simulink model "SimpleVAV"  (R2020a)
settings: Solver=FixedStepAuto  StartTime=0.0  StopTime=7200  RelTol=1e-3
settings Model: Creator=yangyang.fu  LastModifiedBy=yangyang.fu

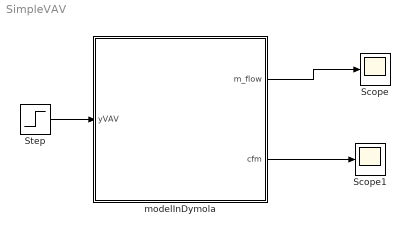
== system SimpleVAV ==
  Scope : Scope
  Scope1 : Scope
  Step : Step  Time=3600  Before=0.5  SampleTime=0.1
  modelInDymola : Subsystem  Tag=07-Sep-2021 15:10:03#975
      mask help:
      | Dymola block.
      | A dymola block allows acausal physical modeling.
      | See Dymola manual for usage.
      settings: CopyFcn=newDymolaGui('07-Sep-2021 15:10:03#975','Copy');  DeleteFcn=if exist('newDymolaGui') newDymolaGui('SimpleVAV/modelInDymola','Delete'); end;  NameChangeFcn=newDymolaGui('07-Sep-2021 15:10:03#975','Copy');  OpenFcn=newDymolaGui('SimpleVAV/modelInDymola','Init');
      mask Display: image(reshape([1;1;1;1;1;1;1;1;1;1;1;1;1;1;1;1;1;1;1;1;1;1;0;0;0;0;0;0;0;0;0;0;1;1;1;1;1;1;1;1;0;1;1;1;1;1;1;1;1;0;1;1;1;1;1;0;0;0;0;0;0;0;1;1;0;0;0;0;0;0;0;1;1;0;0;0;0;0;0;0;1;1;0;0;0;0;0;0;0;1;1;0;0;0;0;0;0;0;1;1;0;0;0;0;0;0;0;1;1;0;0;0;0;0;0;0;1;1;0;0;0;0;0;0;0;1;1;0;0;0;0;0;0;0;1;1;0;0;0;0;0;0;0;1;1;0;0;0;0;0;0;0;1;1;0;0;0;0;0;0;0;1;1;0;0;0;0;0;0;0;1;1;0;0;0;0;0;0;0;1;1;0;0;0;0;0;0;0;1;1;0;0;0;0;0;0;0;1;1;0;0;0;0;0;0;0;1;1;0;0;0;0;0;0;0;1;1;0;0;0;0;0;0;0;1;1;0;0;0;0;0;0;0;1;1;0;0;0;0;0;0;0;1;1;0;0;0;0;0;0;0;1;1;0;0;0;0;0;0;0;1;1;0;0;0;0;0;0;0;1;1;1;1;1;0;1;1;1;1;1;1;1;1;0;1;1;1;1;1;1;1;1;0;0;0;0;0;0;0;0;0;0;1;1;1;1;1;1;1;1;1;1;1;1;1;1;1;1;1;1;1;1;1;1;1;1;1;1;1;1;1;1;1;1;1;1;1;1;1;1;1;1;1;1;1;1;0;0;0;0;0;0;0;0;0;0;1;1;1;1;1;1;1;1;0;1;1;1;1;1;1;1;1;0;1;1;1;1;1;0;0;0;0;0;0;0;1;1;0;0;0;0;0;0;0;1;1;0;0;0;0;0;0;0;1;1;0;0;0;0;0;0;0;1;1;0;0;0;0;0;0;0;1;1;0;0;0;0;0;0;0;1;1;0;0;0;0;0;0;0;1;1;0;0;0;0;0;0;0;1;1;0;0;0;0;0;0;0;1;1;0;0;0;0;0;0;0;1;1;0;0;0;0;0;0;0;1;1;0;0;0;0;0;0;0;1;1;0;0;0;0;0;0;0;1;1;0;0;0;0;0;0;0;1;1;0;0;0;0;0;0;0;1;1;0;0;0;0;0;0;0;1;1;0;0;0;0;0;0;0;1;1;0;0;0;0;0;0;0;1;1;0;0;0;0;0;0;0;1;1;0;0;0;0;0;0;0;1;1;0;0;0;0;0;0;0;1;1;0;0;0;0;0;0;0;1;1;0;0;0;0;0;0;0;1;1;0;0;0;0;0;0;0;1;1;1;1;1;0;1;1;1;1;1;1;1;1;0;1;1;1;1;1;1;1;1;0;0;0;0;0;0;0;0;0;0;1;1;1;1;1;1;1;1;1;1;1;1;1;1;1;1;1;1;1;1;1;1;1;1;1;1;1;1;1;1;1;1;1;1;1;1;1;1;1;1;1;1;1;1;0;0;0;0;0;0;0;0;0;0;1;1;1;1;1;1;1;1;0;1;1;1;1;1;1;1;1;0;1;1;1;1;1;0;0;0;0;0;0;0;1;1;0;0;0;0;0;0;0;1;1;0;1;1;1;1;1;0;1;1;0;1;1;1;1;1;0;1;1;0;1;1;1;1;1;0;1;1;0;1;1;1;1;1;0;1;1;0;1;1;1;1;1;0;1;1;0;1;1;1;1;1;0;1;1;0;1;1;1;1;1;0;1;1;0;1;1;1;1;1;0;1;1;0;1;1;1;1;1;0;1;1;0;1;1;1;1;1;0;1;1;0;1;1;1;1;1;0;1;1;0;1;1;1;1;1;0;1;1;0;1;1;1;1;1;0;1;1;0;1;1;1;1;1;0;1;1;0;1;1;1;1;1;0;1;1;0;1;1;1;1;1;0;1;1;0;1;1;1;1;1;0;1;1;0;1;1;1;1;1;0;1;1;0;1;1;1;1;1;0;1;1;0;1;1;1;1;1;0;1;1;0;0;0;0;0;0;0;1;1;0;0;0;0;0;0;0;1;1;1;1;1;0;1;1;1;1;1;1;1;1;0;1;1;1;1;1;1;1;1;0;0;0;0;0;0;0;0;0;0;1;1;1;1;1;1;1;1;1;1;1;1;1;1;1;1;1;1;1;1;1;1],18,18,3),[.2,.2,.6,.6])
  wires:
  Step/1 -> modelInDymola/1(yVAV)
  modelInDymola/1(m_flow) -> Scope/1
  modelInDymola/2(cfm) -> Scope1/1

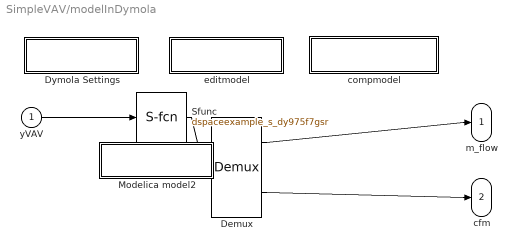
== system SimpleVAV/modelInDymola ==
  yVAV : Inport
  Demux : Demux  Outputs=[1;1]
  Dymola Settings : Subsystem  mask{ModelName=dSpaceExample.SimpleVAV, MoFileName=D:/github/dspace-modelica-example/dSpaceExample/SimpleVAV.mo, dSpace=, BusConnector=[], ResultFile=[], ResultFileOnline=[], ResultDt=[], Libs=:, bigobj=[], ImportFolder=[], guimode=[], ModelName2=[], forRuntime=[], MEXLoad=[], omitDescription=[], ResultName=dspaceexample_s_dy975f7gsr}
      mask prompts: ModelName "Name of Dymola model"; MoFileName "File Name (including .mo)"; ResultFile "Create Result"; ResultFileOnline "Load result"; ResultDt "Result min dt"; Libs "Used Libraries"; bigobj "Compiler flag /bigobj"; ImportFolder "Import folder"; guimode "GUI mode flag"; ModelName2 "Model name for import mode"; forRuntime "Runtime export"; MEXLoad "Compiled S-function"; omitDescription "Omit description strings"; ResultName "Name of result file"
      mask Display: disp('Dymola Settings');
  Modelica model2 : Subsystem
      mask Display: disp('Change parameters');
  Sfunc : S-Function  Tag=975f7gsr  FunctionName=dspaceexample_s_dy975f7gsr  Parameters=[vav_vav_sta_default_p;vav_vav_sta_default_T;vav_vav_sta_default_X;vav_vav_riseTime;vav_vav_y_start;vav_vav_filter_gain;vav_vav_filter_A_ripple;vav_vav_filter_f_min;vav_vav_filter_normalized;vav_vav_filter_x_start;vav_vav_filter_u_nominal;vav_vav_use_deltaM;vav_vav_deltaM;vav_vav_roundDuct;vav_vav_ReC;vav_vav_a;vav_vav_b;vav_vav_yL;vav_vav_yU;vav_vav_k1;vav_vav_l;vav_vav_l2;vav_vav_deltax;vav_vav_y_min;vav_terHea_bal1_preDro_st25;vav_terHea_bal1_preDro_st26;vav_terHea_bal1_preDro_st27;vav_terHea_bal2_preDro_st28;vav_terHea_bal2_preDro_st29;vav_terHea_delta;vav_terHea_T_a1_nominal;vav_terHea_T_a2_nominal;vav_terHea_r_nominal;vav_terHea_hA_n_w;vav_terHea_hA_n_a;vav_terHea_hA_T0_w;vav_terHea_hA_T0_a;vav_sinTer_X;vav_sinTer_p;vav_sinTer_T;vav_souTer_X;vav_souTer_m_flow;vav_souTer_T;zer_k;sou_X;sou_p;sou_T;sin_X;sin_p;sin_T;VRoo;toVol_k],[vav_vav_filter_x]  PortCounts=[1;1]  SFunctionDeploymentMode=off  EnableBusSupport=off  mask{vav_vav_sta_default_p=101325, vav_vav_sta_default_T=293.15, vav_vav_sta_default_X=[0.01; 0.99], vav_vav_riseTime=120, vav_vav_y_start=1, vav_vav_filter_gain=1, vav_vav_filter_A_ripple=0.5, vav_vav_filter_f_min=0, vav_vav_filter_normalized=1, vav_vav_filter_x_start=[0; 0], vav_vav_filter_u_nominal=1, vav_vav_use_deltaM=1, vav_vav_deltaM=0.3, vav_vav_roundDuct=0, vav_vav_ReC=4000, vav_vav_a=-1.51, vav_vav_b=9.45, vav_vav_yL=0.166666666666667, vav_vav_yU=0.611111111111111, vav_vav_k1=0.45, vav_vav_l=0.0001, vav_vav_l2=0.01, vav_vav_deltax=0.02, vav_vav_y_min=0.02, vav_terHea_bal1_preDro_st25=101325, vav_terHea_bal1_preDro_st26=293.15, vav_terHea_bal1_preDro_st27=[0.01; 0.99], vav_terHea_bal2_preDro_st28=300000, vav_terHea_bal2_preDro_st29=293.15, vav_terHea_delta=0.001, vav_terHea_T_a1_nominal=289.85, vav_terHea_T_a2_nominal=355.35, vav_terHea_r_nominal=0.666666666666667, vav_terHea_hA_n_w=0.85, vav_terHea_hA_n_a=0.8, vav_terHea_hA_T0_w=293.15, vav_terHea_hA_T0_a=293.15, vav_sinTer_X=1, vav_sinTer_p=300000, vav_sinTer_T=293.15, vav_souTer_X=1, vav_souTer_m_flow=0, vav_souTer_T=323.15, zer_k=0, sou_X=[0.01; 0.99], sou_p=101565, sou_T=286.15, sin_X=[0.01; 0.99], sin_p=101325, sin_T=293.15, VRoo=2698, toVol_k=1642.54263565891, vav_vav_filter_x=[0; 0]}
      mask prompts: vav_vav_sta_default_p "vav.vav.sta_default.p"; vav_vav_sta_default_T "vav.vav.sta_default.T"; vav_vav_sta_default_X "vav.vav.sta_default.X"; vav_vav_riseTime "vav.vav.riseTime"; vav_vav_y_start "vav.vav.y_start"; vav_vav_filter_gain "vav.vav.filter.gain"; vav_vav_filter_A_ripple "vav.vav.filter.A_ripple"; vav_vav_filter_f_min "vav.vav.filter.f_min"; vav_vav_filter_normalized "vav.vav.filter.normalized"; vav_vav_filter_x_start "vav.vav.filter.x_start"; vav_vav_filter_u_nominal "vav.vav.filter.u_nominal"; vav_vav_use_deltaM "vav.vav.use_deltaM"; vav_vav_deltaM "vav.vav.deltaM"; vav_vav_roundDuct "vav.vav.roundDuct"; vav_vav_ReC "vav.vav.ReC"; vav_vav_a "vav.vav.a"; vav_vav_b "vav.vav.b"; vav_vav_yL "vav.vav.yL"; vav_vav_yU "vav.vav.yU"; vav_vav_k1 "vav.vav.k1"; vav_vav_l "vav.vav.l"; vav_vav_l2 "vav.vav.l2"; vav_vav_deltax "vav.vav.deltax"; vav_vav_y_min "vav.vav.y_min"; vav_terHea_bal1_preDro_st25 "vav.terHea.bal1.preDro.sta_default.p"; vav_terHea_bal1_preDro_st26 "vav.terHea.bal1.preDro.sta_default.T"; vav_terHea_bal1_preDro_st27 "vav.terHea.bal1.preDro.sta_default.X"; vav_terHea_bal2_preDro_st28 "vav.terHea.bal2.preDro.sta_default.p"; vav_terHea_bal2_preDro_st29 "vav.terHea.bal2.preDro.sta_default.T"; vav_terHea_delta "vav.terHea.delta"; vav_terHea_T_a1_nominal "vav.terHea.T_a1_nominal"; vav_terHea_T_a2_nominal "vav.terHea.T_a2_nominal"; vav_terHea_r_nominal "vav.terHea.r_nominal"; vav_terHea_hA_n_w "vav.terHea.hA.n_w"; vav_terHea_hA_n_a "vav.terHea.hA.n_a"; vav_terHea_hA_T0_w "vav.terHea.hA.T0_w"; vav_terHea_hA_T0_a "vav.terHea.hA.T0_a"; vav_sinTer_X "vav.sinTer.X"; vav_sinTer_p "vav.sinTer.p"; vav_sinTer_T "vav.sinTer.T"; vav_souTer_X "vav.souTer.X"; vav_souTer_m_flow "vav.souTer.m_flow"; vav_souTer_T "vav.souTer.T"; zer_k "zer.k"; sou_X "sou.X"; sou_p "sou.p"; sou_T "sou.T"; sin_X "sin.X"; sin_p "sin.p"; sin_T "sin.T"; toVol_k "toVol.k"; vav_vav_filter_x "vav.vav.filter.x"
      mask Display: image(imread('Dymola.bmp'))
  compmodel : Subsystem
      settings: OpenFcn=compileModelica('SimpleVAV/modelInDymola');
      mask Display: disp('Compile Modelica model');
  editmodel : Subsystem
      settings: OpenFcn=editModelica('SimpleVAV/modelInDymola');
      mask Display: disp('Edit Modelica model');
  m_flow : Outport
  cfm : Outport  Port=2
  wires:
  Sfunc/1 -> Demux/1
  Demux/1 -> m_flow/1
  Demux/2 -> cfm/1
  yVAV/1 -> Sfunc/1

== system SimpleVAV/modelInDymola/Dymola Settings ==

== system SimpleVAV/modelInDymola/Modelica model2 ==

== system SimpleVAV/modelInDymola/compmodel ==

== system SimpleVAV/modelInDymola/editmodel ==
